simulink model "Pacuraru_Fabian_Lab3"  (R2013b)
settings: Solver=ode45  StartTime=0.0  StopTime=10.0  MaxStep=0.0005  RelTol=1e-3
libraries: powerlib x5
settings Model: Creator=Student  LastModifiedBy=Student

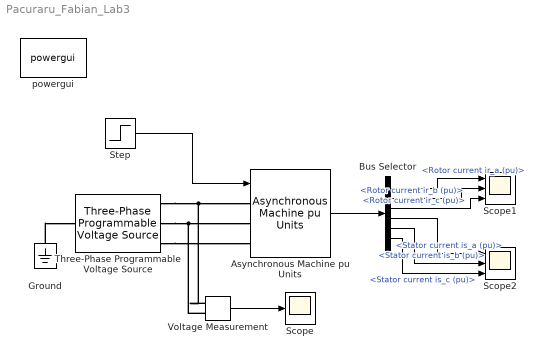
== system Pacuraru_Fabian_Lab3 ==
  Asynchronous Machine pu Units : powerlib/Machines/Asynchronous Machine pu Units  PresetModel=No  MechanicalLoad=Torque Tm  ShowDetailedParameters=on  RotorType=Squirrel-cage  ReferenceFrame=Rotor  NominalParameters=[3730 460 60]  Stator=[0.01965 0.0397]  Rotor=[0.01909 0.0397]  Cage1=[0.01909 0.0397]  Cage2=[0.01909 0.0397]  Lm=1.354  Mechanical=[0.09526 0.05479 2]  PolePairs=2  InitialConditions=[0 0 0 0 0 0 0 0]  Units=pu  LoadFlowParameters=0  SimulateSaturation=off  Saturation="[0.212,0.4201,0.8125,1.0979,1.4799,2.2457,3.2586,4.5763,6.4763 ;   0.5,0.7,0.9,1,1.1,1.2 ,1.3,1.4,1.5]"  TsPowergui=0  TsBlock=-1  IterativeModel=Trapezoidal non iterative  Pmec=0
  Bus Selector : BusSelector  OutputSignals=Rotor measurements.Rotor current ir_a (pu),Rotor measurements.Rotor current ir_b (pu),Rotor measurements.Rotor current ir_c (pu),Stator measurements.Stator current is_a (pu),Stator measurements.Stator current is_b (pu),Stator measurements.Stator current is_c (pu)
  Ground : powerlib/Elements/Ground  LConnTagsString=a
  Scope : Scope
  Scope1 : Scope  NumInputPorts=3
      settings: YMin=-5~-5~-5  YMax=5~5~5
  Scope2 : Scope  NumInputPorts=3
      settings: YMin=-5~-5~-5  YMax=5~5~5  SaveName=ScopeData2
  Step : Step  Time=6  After=10  SampleTime=0
  Three-Phase Programmable Voltage Source : powerlib/Electrical Sources/Three-Phase Programmable Voltage Source  PositiveSequence=[400 0 50]  VariationEntity=Amplitude  VariationType=Table of time-amplitude pairs  VariationTypeAlt=Step  VariationStep=0.5  VariationRate=10  VariationMagnitude=0.3  VariationFrequency=2  VariationTiming=[1 2]  VariationPhaseA=off  Amplitudes=[0 1 0 1]  TimeValues=[0 0.5 1.2 1.4]  HarmonicGeneration=off  HarmonicA=[3 0.2 -25 0]  HarmonicB=[2 0.15 35 2]  Timing="[0.05  3]"  BusType=swing  Pref=0  Qref=0  Qmin=-inf  Qmax=inf
  Voltage Measurement : powerlib/Measurements/Voltage Measurement  PhasorSimulation=off  OutputType=Complex  PSBequivalent=0
  powergui : powerlib/powergui  Priority=1  SimulationMode=Continuous  SolverType=Tustin  SampleTime=50e-6  frequency=60  SPID=off  DisableSnubberDevices=off  DisableRonSwitches=off  DisableVfSwitches=off  SwTol=0  Interpol=off  DisplayEquations=off  frequencyindice=60  Pbase=100e6  ErrMax=1e-4  Iterations=50  UnitsV=kV  UnitsW=MW  FunctionMessages=off  echomessages=off  HookPort=off  EnableUseOfTLC=off  x0status=blocks  RestoreLinks=warning  ResistiveCurrentMeasurement=off  Frange=[0:2:500]  Ylog=off  Xlog=on  ShowGrid=off  save=off  variable=ZData  ZoomFFT=off  StartTime=0.0  cycles=1  DisplayStyle=1  fundamental=60  FreqAxis=off  MaxFrequency=1000  frequencyindicesteady=1  RmsSteady=1  display=off  Ts=0  methode=off
  wires:
  Step/1 -> Asynchronous Machine pu Units/1
  Asynchronous Machine pu Units/1 -> Bus Selector/1
  Voltage Measurement/1 -> Scope/1
  Bus Selector/1 -> Scope1/1  "<Rotor current ir_a (pu)>"
  Bus Selector/2 -> Scope1/2  "<Rotor current ir_b (pu)>"
  Bus Selector/3 -> Scope1/3  "<Rotor current ir_c (pu)>"
  Bus Selector/4 -> Scope2/1  "<Stator current is_a (pu)>"
  Bus Selector/5 -> Scope2/2  "<Stator current is_b (pu)>"
  Bus Selector/6 -> Scope2/3  "<Stator current is_c (pu)>"
  connections:
  Three-Phase Programmable Voltage Source/RConn1 -- Voltage Measurement/LConn1 -- Asynchronous Machine pu Units/LConn1
  Three-Phase Programmable Voltage Source/RConn2 -- Voltage Measurement/LConn2 -- Asynchronous Machine pu Units/LConn2
  Three-Phase Programmable Voltage Source/RConn3 -- Asynchronous Machine pu Units/LConn3
  Ground/LConn1 -- Three-Phase Programmable Voltage Source/LConn1
